simulink model "disturbance_simulation"  (R2020a)
settings: Solver=FixedStepAuto  StartTime=0.0  StopTime=100  FixedStep=0.01  RelTol=1e-3  EnableMultiTasking=on
values from neighbouring files (symbols this model uses):
  E_b_ECI_0 = rotm2eul(C_b_ECI_0)    [Disturbance_Initial.m]
  orbit0 = [r_ECI_0'; v_ECI_0']    [Disturbance_Initial.m]
  sun_ECI = [1; 0; 0]    [Disturbance_Initial.m]
  surfaceProperties = [Areas cps normals]    [Disturbance_Initial.m]
  w_b_ECI_0 = [0.001; -0.001; 0.002]    [Disturbance_Initial.m]
undefined symbols (not defined in the file or in its folder): IAU
libraries: aerolibtransform2 x1
settings Model: SimulationMode=external  Creator=sheab  LastModifiedBy=sheab
settings SolverCC: ConcurrentTasks=on  AutoInsertRateTranBlk=on
settings DataIOCC: SaveFormat=StructureWithTime
settings OptimizationCC: BlockReduction=off  OptimizeBlockIOStorage=off
settings DebuggingCC: UnderSpecifiedDataTypeMsg=warning  UnconnectedInputMsg=none  UnconnectedOutputMsg=none  UnconnectedLineMsg=none  UnderSpecifiedDimensionMsg=warning
settings HardwareCC: ProdBitPerPointer=32  ProdBitPerSizeT=32  ProdBitPerPtrDiffT=32  ProdLargestAtomicFloat=None  ProdWordSize=32  ProdLongLongMode=on  ProdHWDeviceType=Generic->32-bit x86 compatible
settings ModelReferenceCC: EnableRefExpFcnMdlSchedulingChecks=off
settings RTWCC: Description=Simulink Real-Time  SystemTargetFile=slrt.tlc  TemplateMakefile=slrt_default_tmf  CodeExecutionProfiling=on  RTWCompilerOptimization=on
settings SimulinkRealTimeCC: SupportVariableSizeSignals=on  RL32LogTETModifier=off  xPCConcurrentTasks=on

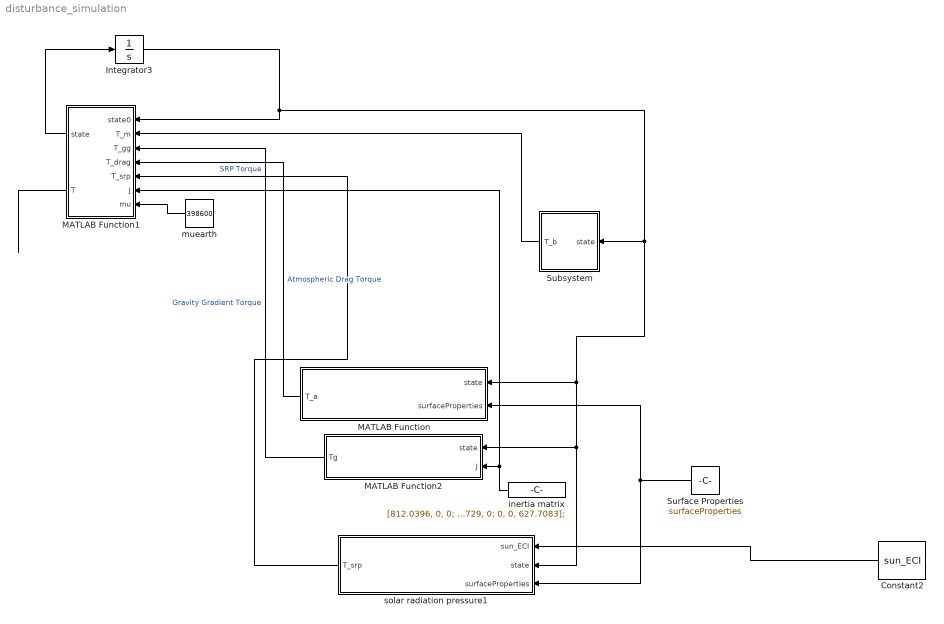
== system disturbance_simulation ==
  Constant2 : Constant  Value=sun_ECI
  Integrator3 : Integrator  InitialCondition=[w_b_ECI_0; E_b_ECI_0'; q_b_ECI_0'; orbit0]
  MATLAB Function : MATLAB Function  TreatAsAtomicUnit=on
  MATLAB Function1 : MATLAB Function  TreatAsAtomicUnit=on
  MATLAB Function2 : MATLAB Function  TreatAsAtomicUnit=on
  Subsystem : Subsystem
  Surface Properties : Constant  Value=surfaceProperties  VectorParams1D=off
  inertia matrix : Constant  Value=[812.0396, 0, 0; 0, 545.3729, 0; 0, 0, 627.7083];  VectorParams1D=off
  muearth : Constant  Value=398600  VectorParams1D=off
  solar radiation pressure1 : MATLAB Function  TreatAsAtomicUnit=on
  wires:
  inertia matrix/1 -> MATLAB Function2/2(J), MATLAB Function1/6(J)
  solar radiation pressure1/1(T_srp) -> MATLAB Function1/5(T_srp)  "SRP Torque"
  muearth/1 -> MATLAB Function1/7(mu)
  MATLAB Function2/1(Tg) -> MATLAB Function1/3(T_gg)  "Gravity Gradient Torque"
  MATLAB Function/1(T_a) -> MATLAB Function1/4(T_drag)  "Atmospheric Drag Torque"
  Constant2/1 -> solar radiation pressure1/1(sun_ECI)
  Surface Properties/1 -> MATLAB Function/2(surfaceProperties), solar radiation pressure1/3(surfaceProperties)
  MATLAB Function1/2(T) -> ?
  Integrator3/1 -> MATLAB Function1/1(state0), solar radiation pressure1/2(state), MATLAB Function2/1(state), MATLAB Function/1(state), Subsystem/1(state)
  MATLAB Function1/1(state) -> Integrator3/1
  Subsystem/1(T_b) -> MATLAB Function1/2(T_m)

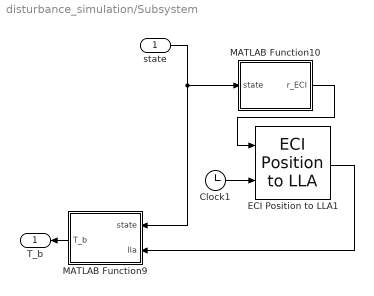
== system disturbance_simulation/Subsystem ==
  state : Inport
  Clock1 : Clock
  ECI Position to LLA1 : aerolibtransform2/ECI Position to LLA  red=IAU-2000/2006  year=2020  month=March  day=20  hour=12  min=0  sec=0  deltaT=Sec  errorflag=Error  extraparamflag=off  eunits=Metric (MKS)  earthmodel=WGS84  flat=1/298.257223563  eqradius=6378137
      settings: AttributesFormatString=%<red>  SourceProductBaseCode=AE
  MATLAB Function10 : MATLAB Function  TreatAsAtomicUnit=on
  MATLAB Function9 : MATLAB Function  TreatAsAtomicUnit=on
  T_b : Outport
  wires:
  state/1 -> MATLAB Function10/1(state), MATLAB Function9/1(state)
  Clock1/1 -> ECI Position to LLA1/2
  ECI Position to LLA1/1 -> MATLAB Function9/2(lla)
  MATLAB Function10/1(r_ECI) -> ECI Position to LLA1/1
  MATLAB Function9/1(T_b) -> T_b/1

== matlab function disturbance_simulation/MATLAB Function1 ==
  data: state0 input; state output; T_m input; T_gg input; T_drag input; T_srp input; J input; mu input; T output
function [state, T] = attitude(state0, T_m, T_gg, T_drag, T_srp, J, mu)

% initial state
w = [state0(1); state0(2); state0(3)];
wx = [0, -w(3), w(2); w(3), 0, -w(1); -w(2), w(1), 0]; % omega cross
 epsilon = [state0(7); state0(8); state0(9)];
epsilonx = [0, -epsilon(3), epsilon(2); epsilon(3), 0, -epsilon(1); -epsilon(2), epsilon(1), 0]; % epsilon cross
 eta = state0(10);
 phi = state0(4);
 theta = state0(5);
 psi = state0(6);

T = T_m + T_gg + T_drag + T_srp;

%derivatives
wp = J^(-1)*(T - wx*J*w);
epsilonp = 0.5*(eta*eye(3) + epsilonx)*w;
etap = -0.5*epsilon'*w; % derivative of eta

Ep = (1/cos(theta))*[cos(theta), sin(phi)*sin(theta), cos(phi)*sin(theta); ...
                          0, cos(phi)*cos(theta), -sin(phi)*cos(theta); ...
                          0, sin(phi), cos(phi)];

Ep = Ep*w;

% initial state
rx = state0(11);
ry = state0(12);
rz = state0(13);
r = [rx; ry; rz];

rxp = state0(14);
ryp = state0(15);
rzp = state0(16);
rp = [rxp; ryp; rzp];

rxpp = -mu*rx/norm(r)^3;
rypp = -mu*ry/norm(r)^3;
rzpp = -mu*rz/norm(r)^3;
rpp = [rxpp; rypp; rzpp];

rv_dot = [rp; rpp];

state = [wp; Ep; epsilonp; etap; rv_dot];

end

== matlab function disturbance_simulation/MATLAB Function ==
  data: state input; T_a output; surfaceProperties input
function T_a  = atmosdrag(state, surfaceProperties)
q_b_ECI = [state(10); state(7); state(8); state(9)];
r_ECI = [state(11); state(12); state(13)];
v_ECI = [state(14); state(15); state(16)];

v_b = quat2rotm(q_b_ECI')*v_ECI;
Cd = 2.1;
Re = 6378.137;

rho_0 = 3.614e-14;
H = 88.667;
h_0 = 700;
nr = sqrt(r_ECI(1)^2 + r_ECI(2)^2 + r_ECI(3)^2);

density = rho_0*exp(-(nr - Re - h_0)/H);
T_a = zeros([3,1]);

nv = sqrt(v_ECI(1)^2 + v_ECI(2)^2 + v_ECI(3)^2);

for i = 1:length(surfaceProperties)
    A = surfaceProperties(i,1);
    cp = surfaceProperties(i,2:4);
    n = surfaceProperties(i,5:7);
    wet = n*v_b/sqrt(v_b(1)^2 + v_b(2)^2 + v_b(3)^2);
    if wet > 0
        A_wet = A*wet;
        v_b_hat = v_b/sqrt(v_b(1)^2 + v_b(2)^2 + v_b(3)^2);
        F_a = -1/2*density*(nv*1000)^2*Cd*A_wet*v_b_hat;
        T_a = T_a + cross(cp', F_a);
    end
end

== matlab function disturbance_simulation/solar radiation pressure1 ==
  data: sun_ECI input; state input; surfaceProperties input; T_srp output
function T_srp = srp(sun_ECI, state, surfaceProperties)
% solar pressure (SRP)

p_sun = 4.5e-6; %N/m
q_b_ECI = [state(10); state(7); state(8); state(9)];

sun_b = quat2rotm(q_b_ECI')*sun_ECI;
T_srp = zeros([3,1]);
ns = sqrt(sun_b(1)^2 + sun_b(2)^2 + sun_b(3)^2);

%rho_sum = zeros([3,1]);
% Solar Radiation Pressure
for i = 1:length(surfaceProperties)
    A = surfaceProperties(i,1);
    cp = surfaceProperties(i,2:4);
    n = surfaceProperties(i,5:7);
    wet = n*sun_b/ns;
    if wet > 0
        A_wet = A*wet;
        F_srp = p_sun*A_wet*sun_b;
        T_srp = T_srp + cross(cp', F_srp);
        %rho_sum = rho_sum + rho';
    end
end

== matlab function disturbance_simulation/MATLAB Function2 ==
  data: state input; Tg output; J input
function Tg = gravgrad(state, J)
muearth = 398600;

q_b_ECI = [state(10); state(7); state(7); state(9)];
r_ECI = [state(11); state(12); state(13)];

r_b = quat2rotm(q_b_ECI')*r_ECI;
r_b_x = [0, -r_b(3), r_b(2); r_b(3), 0, -r_b(1); -r_b(2), r_b(1), 0];

Tg = 3*muearth/sqrt(r_b(1)^2 + r_b(2)^2 + r_b(3)^2)^5*r_b_x*J*r_b;

end

== matlab function disturbance_simulation/Subsystem/MATLAB Function10 ==
  data: state input; r_ECI output
function r_ECI = postion(state)

r_ECI = [state(11); state(12); state(13)];

== matlab function disturbance_simulation/Subsystem/MATLAB Function9 ==
  data: state input; T_b output; lla input
function T_b = wmm(state, lla)
m_b = 0.5*[0;0;-1];
m_bx = [0, -m_b(3), m_b(2); m_b(3), 0, -m_b(1); -m_b(2), m_b(1), 0];

%JD0 = 2458929.0;

%JD = JD0 + t/(24*3600);

a = 6371.2;
g_11 = -1450.9;
h_11 = 4652.5;
g_10 = -29404.8;

m_ECEF = a^3*[g_11; h_11; g_10];
m_ECEF = m_ECEF*1e-9*1000^3;

r_ECI = [state(11); state(12); state(13)]*1000;
r = norm(r_ECI);

long = lla(2);
angle = (-long*pi/180);
Cz = [cos(angle), -sin(angle), 0; sin(angle), cos(angle), 0; 0, 0, 1];

m_ECI = Cz*m_ECEF;

B_ECI = (3*m_ECI'*r_ECI*r_ECI - r^2*m_ECI)/r^5;

C_b_ECI = quat2rotm([state(10), state(7), state(8), state(9)]);

B_b = C_b_ECI*B_ECI;

T_b = m_bx*B_b;
